simulink model "controller"  (Simulink 7.7)
settings: Solver=FixedStepDiscrete  StartTime=0.0  StopTime=inf  RelTol=1e-3
InitFcn:
  | initRov14;
values from neighbouring files (symbols this model uses):
  fake = eye(12)    [initRov14.m]
  k = [ 20   5   15 ... (first row only)    [initRov14.m]    (also in initSharedMem.m = [ 0*20   0*5   0*15)
undefined symbols (not defined in the file or in its folder): DiscIntNeverNeededParam
libraries: WBCLibrary x16, simulink x2, dspsigops x2
settings Model: Creator=daniele  LastModifiedBy=jorhabib
settings DataIOCC: SignalLoggingSaveFormat=Dataset
settings DebuggingCC: FcnCallInpInsideContextMsg=Enable All

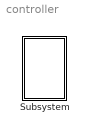
== system controller ==
  Subsystem : Subsystem  mask{robotName='icubGazeboSim', Ts=0.01, localName='dynamicBalancing'}
      mask prompts: robotName "robot name"; localName "module name"

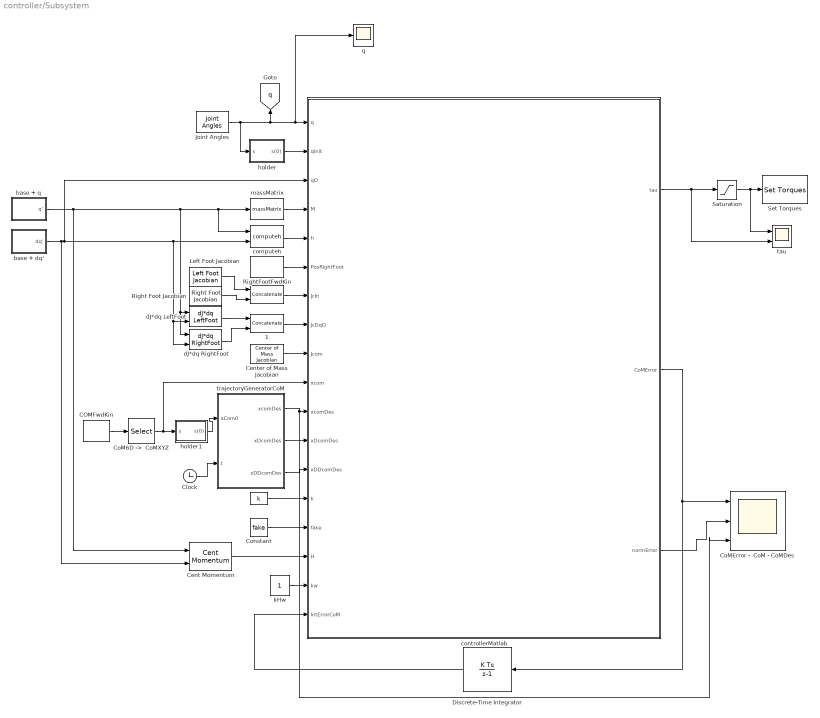
== system controller/Subsystem ==
  "    " : Constant  Value=k
  " " : Concatenate  Mode=Multidimensional array
  " 1" : Concatenate  Mode=Multidimensional array
  "COMFwdKin " : WBCLibrary/wholeBodyModel/Forward Kinematics/COMFwdKin   robotName=robotName  localName=localName
  Cent Momentum : WBCLibrary/wholeBodyModel/Dynamics/Cent Momentum  robotName=robotName  localName=localName
  Center of Mass Jacobian : WBCLibrary/wholeBodyModel/Jacobians/Center of Mass Jacobian  robotName=robotName  localName=localName
  Clock : Clock
  "CoM6D ->  CoMXYZ" : Selector  InputPortWidth=7  IndexOptions=Index vector (dialog)  Indices=[1 2 3]  OutputSizes=1
  "CoMError -  CoM - CoMDes " : Scope  NumInputPorts=3
      settings: TimeRange=70  YMin=-0.2~-0.125~-0.1  YMax=0.15~0.45~0.6000000000000001  SaveName=ScopeData6
  Constant : Constant  Value=fake
  Discrete-Time Integrator : DiscreteIntegrator  SampleTime=Ts  ICPrevOutput=DiscIntNeverNeededParam  ICPrevScaledInput=DiscIntNeverNeededParam
  Joint Angles : WBCLibrary/wholeBodyStates/Joint Angles  robotName=robotName  localName=localName
  Left Foot Jacobian : WBCLibrary/wholeBodyModel/Jacobians/Left Foot Jacobian  robotName=robotName  localName=localName
  Right Foot Jacobian : WBCLibrary/wholeBodyModel/Jacobians/Right Foot Jacobian  robotName=robotName  localName=localName
  RightFootFwdKin : WBCLibrary/wholeBodyModel/Forward Kinematics/RightFootFwdKin  robotName=robotName  localName=localName
  Saturation : Saturate  UpperLimit=40  LowerLimit=-40  SampleTime=Ts
  Set Torques : WBCLibrary/wholeBodyActuators/Set Torques  val=6  robotName=robotName  localName=localName
  base + dq' : Subsystem
  base + q : Subsystem
  computeh : WBCLibrary/wholeBodyModel/Dynamics/computeh  val=7  robotname=robotName  localname=localName
  controllerMatlab : Stateflow chart  TreatAsAtomicUnit=on
      settings: PermitHierarchicalResolution=ParametersOnly
  dJ*dq LeftFoot : WBCLibrary/wholeBodyModel/Dynamics/dJ*dq LeftFoot  val=9  robotName=robotName  localName=localName
  dJ*dq RightFoot : WBCLibrary/wholeBodyModel/Dynamics/dJ*dq RightFoot  val=9  robotName=robotName  localName=localName
  holder : Subsystem
  holder1 : Subsystem
  kHw : Constant
  massMatrix : WBCLibrary/wholeBodyModel/Dynamics/massMatrix  val=8  robotname=robotName  localname=localName
  q : Scope
      settings: YMin=-20  YMax=20
  tau : Scope  NumInputPorts=2
      settings: YMin=-20~-30  YMax=20~30  SaveName=ScopeData4
  trajectoryGeneratorCoM : Stateflow chart  TreatAsAtomicUnit=on
      settings: PermitHierarchicalResolution=ParametersOnly
  tag scope: q=global
  wires:
  computeh/1 -> controllerMatlab/5(h)
  massMatrix/1 -> controllerMatlab/4(M)
  Joint Angles/1 -> holder/1(s), [q], q/1, controllerMatlab/1(q)
  Center of Mass Jacobian/1 -> controllerMatlab/9(Jcom)
  "    "/1 -> controllerMatlab/14(k)
  Left Foot Jacobian/1 -> " "/1
  Right Foot Jacobian/1 -> " "/2
  trajectoryGeneratorCoM/1(xcomDes) -> "CoMError -  CoM - CoMDes "/3, controllerMatlab/11(xcomDes)
  trajectoryGeneratorCoM/2(xDcomDes) -> controllerMatlab/12(xDcomDes)
  trajectoryGeneratorCoM/3(xDDcomDes) -> controllerMatlab/13(xDDcomDes)
  Clock/1 -> trajectoryGeneratorCoM/2(t)
  holder1/1(s(0)) -> trajectoryGeneratorCoM/1(xCom0)
  dJ*dq LeftFoot/1 -> " 1"/1
  dJ*dq RightFoot/1 -> " 1"/2
  "COMFwdKin "/1 -> "CoM6D ->  CoMXYZ"/1
  "CoM6D ->  CoMXYZ"/1 -> holder1/1(s), controllerMatlab/10(xcom)
  holder/1(s(0)) -> controllerMatlab/2(qInit)
  controllerMatlab/1(tau) -> tau/2, Saturation/1
  RightFootFwdKin/1 -> controllerMatlab/6(PosRightFoot)
  controllerMatlab/2(CoMError) -> Discrete-Time Integrator/1, "CoMError -  CoM - CoMDes "/1
  Discrete-Time Integrator/1 -> controllerMatlab/18(IntErrorCoM)
  Saturation/1 -> tau/1, Set Torques/1
  base + q/1(q') -> computeh/1, massMatrix/1, dJ*dq RightFoot/1, dJ*dq LeftFoot/1, Cent Momentum/1
  base + dq'/1(dq') -> controllerMatlab/3(qD), computeh/2, dJ*dq RightFoot/2, dJ*dq LeftFoot/2, Cent Momentum/2
  Cent Momentum/1 -> controllerMatlab/16(H)
  kHw/1 -> controllerMatlab/17(kw)
  Constant/1 -> controllerMatlab/15(fake)
  controllerMatlab/3(normError) -> "CoMError -  CoM - CoMDes "/2
  " 1"/1 -> controllerMatlab/8(JcDqD)
  " "/1 -> controllerMatlab/7(JcIn)

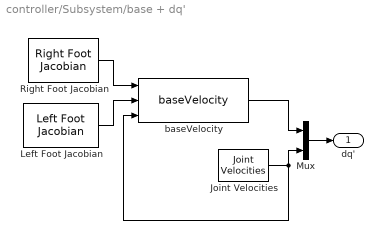
== system controller/Subsystem/base + dq' ==
  Joint Velocities : WBCLibrary/wholeBodyStates/Joint Velocities  robotName=robotName  localName=localName
  Left Foot Jacobian : WBCLibrary/wholeBodyModel/Jacobians/Left Foot Jacobian  robotName=robotName  localName=localName
  Mux : Mux  Inputs=2
  Right Foot Jacobian : WBCLibrary/wholeBodyModel/Jacobians/Right Foot Jacobian  robotName=robotName  localName=localName
  baseVelocity : WBCLibrary/Utilities/baseVelocity
  dq' : Outport
  wires:
  Left Foot Jacobian/1 -> baseVelocity/2
  Right Foot Jacobian/1 -> baseVelocity/1
  baseVelocity/1 -> Mux/1
  Joint Velocities/1 -> baseVelocity/3, Mux/2
  Mux/1 -> dq'/1

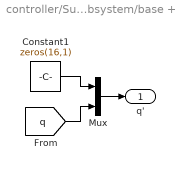
== system controller/Subsystem/base + q ==
  Constant1 : Constant  Value=zeros(16,1)
  Mux : Mux  Inputs=2
  q' : Outport
  wires:
  Mux/1 -> q'/1
  [q] -> Mux/2
  Constant1/1 -> Mux/1

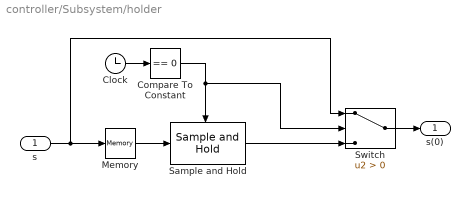
== system controller/Subsystem/holder ==
  s : Inport
  Clock : Clock
  Compare To Constant : simulink/Logic and Bit Operations/Compare To Constant  relop===  const=0  LogicOutDataTypeMode=boolean
  Memory : Memory
  Sample and Hold : dspsigops/Sample and Hold  trig=Falling edge  initCond=0  latchinput=off
  Switch : Switch  Criteria=u2 > Threshold
  s(0) : Outport
  wires:
  s/1 -> Switch/1, Memory/1
  Clock/1 -> Compare To Constant/1
  Compare To Constant/1 -> Sample and Hold/Trigger, Switch/2
  Sample and Hold/1 -> Switch/3
  Switch/1 -> s(0)/1
  Memory/1 -> Sample and Hold/1

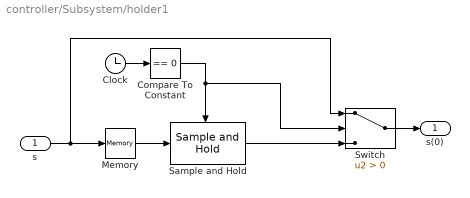
== system controller/Subsystem/holder1 ==
  s : Inport
  Clock : Clock
  Compare To Constant : simulink/Logic and Bit Operations/Compare To Constant  relop===  const=0  LogicOutDataTypeMode=boolean
  Memory : Memory
  Sample and Hold : dspsigops/Sample and Hold  trig=Falling edge  initCond=0  latchinput=off
  Switch : Switch  Criteria=u2 > Threshold
  s(0) : Outport
  wires:
  s/1 -> Switch/1, Memory/1
  Clock/1 -> Compare To Constant/1
  Compare To Constant/1 -> Sample and Hold/Trigger, Switch/2
  Sample and Hold/1 -> Switch/3
  Switch/1 -> s(0)/1
  Memory/1 -> Sample and Hold/1

== matlab function Subsystem/trajectoryGeneratorCoM ==
  data: xcomDes output double; xDcomDes output double; xDDcomDes output double; xCom0 input double; t input double
function [xcomDes, xDcomDes, xDDcomDes] = fcn(xCom0,t)
%#codegen

e3 = [0;1;0];
A = 0.1;
f = 0.1;
t = t*0.8;
% xcomDes    = [xCom0(1:2); (1/A-1)*A*xCom0(3)] + A*xCom0(3)*cos(2*pi*f*t)*e3;
% xDcomDes   = -xCom0(3)*A*2*pi*f*sin(2*pi*f*t)*e3;
% xDDcomDes  = -xCom0(3)*A*(2*pi*f)^2*cos(2*pi*f*t)*e3;

xcomDes    = xCom0 + A*sin(2*pi*f*t)*e3;
xDcomDes   =         A*2*pi*f*cos(2*pi*f*t)*e3;
xDDcomDes  =        -A*(2*pi*f)^2*sin(2*pi*f*t)*e3;

== matlab function Subsystem/controllerMatlab ==
  data: q input double; qInit input double; qD input double; M input double; h input double; PosRightFoot input double; JcIn input double; JcDqD input double; tau output double; Jcom input double; xcom input double; xcomDes input double; xDcomDes input double; xDDcomDes input double; k input double; fake input double; H input double; kw input double; CoMError output double; IntErrorCoM input double; normError output double
function [tau,CoMError,normError] = fcn(q,qInit, qD, M, h, PosRightFoot, JcIn, JcDqD, Jcom, xcom, xcomDes, xDcomDes, xDDcomDes, k, fake, H, kw,IntErrorCoM)
%#codegen

PINV_TOL = 1e-5;
g        = 9.81;

n = size(fake, 1);

DL = 25-n;            %DeltaIndexOnlyLegs

if DL ~= 0
   Jc = [JcIn(:,1:6),JcIn(:,7 + DL:end)]; 
else
   Jc = JcIn; 
end

m     = M(1,1);
Mb    = M(1:6,1:6);
MbInv = inv(Mb);
Mbj   = M(1:6,7 + DL :end); 
Mj    = M(7 + DL :end,7 + DL:end);
U     = [eye(6) , zeros(6,n)];
Jcb   = Jc*U';
SBar  = [  -MbInv*Mbj 
           eye(n)      ];
NjInv = Mj - Mbj'*MbInv*Mbj;

grav = [zeros(2,1);-m*g;zeros(3,1)];

JcSBar     = Jc*SBar;
JcSBarPinv = pinv(JcSBar, PINV_TOL);

% Definition of reference accelerations for CoM and Joints that ensure
% stabilization of desired trajectories xDcomDes and qDes 

xDcom      = Jcom(1:3,:)*qD;
xDDcomStar = xDDcomDes - k(1,1)*(xcom - xcomDes) - k(1,2)*IntErrorCoM - k(1,3)*(xDcom - xDcomDes)  ;
q_starIn   =           - k(2,1)*(q - qInit)                            - k(2,3)*qD(7:end);
if DL ~= 0
   q_star = q_starIn(DL+1:end); 
else
   q_star = q_starIn;
    
end
Pr =  PosRightFoot(1:3) - xcom; % Application point of the contact force on the right foot w.r.t. CoM
A  = [ eye(3),   zeros(3),eye(3), zeros(3);
      -Sf(xcom),  eye(3), Sf(Pr), eye(3) ];

% The following expressions for Ic and IcD hold only if the control 
% objective is the stabilization of the CoM's position
% kw = 0.1;
hwDotDes = H(4:end);
hDotDes = [ m*xDDcomStar ;
            -kw*hwDotDes  ]; 

fd = pinv(A)*(hDotDes-grav);

LambdaStar = JcSBarPinv*(Jcb*MbInv*(h(1:6) - Jcb'*fd) - JcDqD);

NP0 = eye(n) - JcSBarPinv*JcSBar;

LambdaStar = LambdaStar + NP0 * q_star;

tauLegs = - JcSBar'*fd + NjInv*LambdaStar + SBar'*[h(1:6);h(DL + 7:end)];

if DL >= 1 
   tau = h(7:end) - k(3,1)*(q - qInit) - k(3,3)*qD(7:end);   
   tau(DL+1:end) = tauLegs;
else
    tau = tauLegs;
end

CoMError    = xcom - xcomDes;
normError   = norm(CoMError);
